simulink model "ABS_default"  (R2020b)
settings: Solver=VariableStepAuto  StartTime=0.0  StopTime=60.0  RelTol=1e-3
InitFcn:
  | T_B = 0.1;
  | J = 1.13;
  | g = 9.81;
  | road_coeff = [
  |                 1.2801 23.990 0.5200
  |                 0.8570 33.822 0.3470
  |                 1.1973 25.168 0.5373
  |                 0.4004 33.708 0.1204
  |                 0.1946 94.129 0.0646
  |                 0.0500 306.39 0.0010
  |               ];
  | load('ANFIS.mat','train_fis');
  | ce = road_coeff(sel,:);
values from neighbouring files (symbols this model uses):
  Kpid = actSelGen(i,:)    [ABS_ga.m]    (also in ABS_pso.m = Swarm.Particles(k).X)
undefined symbols (not defined in the file or in its folder): m, R, v_x
libraries: fuzblock x1, pid_lib x1
settings Model: Creator=hadlaczkyb  LastModifiedBy=hadlaczkyb
settings DataIOCC: ReturnWorkspaceOutputs=off
settings DebuggingCC: ArithmeticOperatorsInVariantConditions=warning
settings SFSimCC: SimUseLocalCustomCode=off  CustomCodeUndefinedFunction=UseInterfaceOnly
settings RTWCC: RTWUseLocalCustomCode=off

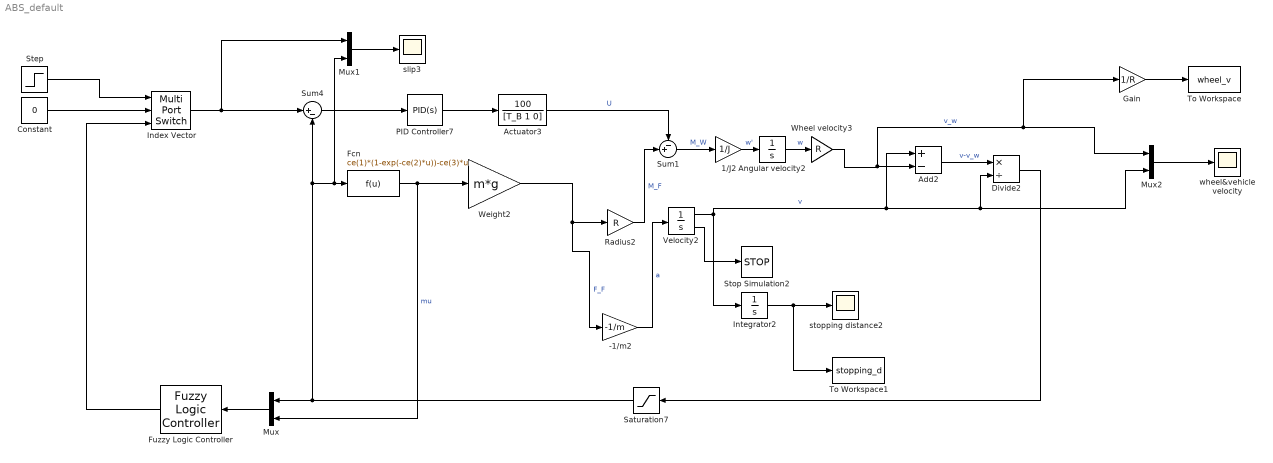
== system ABS_default ==
  -1/m2 : Gain  Gain=-1/m
  1/J2 : Gain  Gain=1/J
  Actuator3 : TransferFcn  Numerator=[0 0 100]  Denominator=[T_B 1 0]
  Add2 : Sum  Inputs=+-
  Angular velocity2 : Integrator  InitialCondition=v_x/R  LimitOutput=on  UpperSaturationLimit=1000  LowerSaturationLimit=0
  Constant : Constant  Value=0
  Divide2 : Product  Inputs=*/
  Fcn : Fcn  Expr=ce(1)*(1-exp(-ce(2)*u))-ce(3)*u
  Fuzzy Logic Controller : fuzblock/Fuzzy Logic  Controller  FIS=train_fis  OutputSampleNumber=101  DataType=double  FuzzifiedInputs=off  RuleFiringStrengths=off  RuleOutputs=off  AggregatedOutputs=off  SimulateUsing=Interpreted execution  OutOfRangeInputValueMessage=warning  NoRuleFiredMessage=warning  EmptyOutputFuzzySetMessage=warning
  Gain : Gain  Gain=1/R
  Index Vector : MultiPortSwitch  DataPortOrder=Zero-based contiguous  Inputs=2  zeroidx=on
  Integrator2 : Integrator
  Mux : Mux  Inputs=2
  Mux1 : Mux  Inputs=2
  Mux2 : Mux  Inputs=2
  PID Controller7 : pid_lib/PID Controller  Controller=PID  Form=Parallel  TimeDomain=Continuous-time  UseExternalTs=off  SampleTime=-1  IntegratorMethod=Forward Euler  FilterMethod=Forward Euler  ControllerParametersSource=internal  P=Kpid(1)  I=Kpid(2)  D=Kpid(3)  UseFilter=on  N=1000  TunerSelectOption=Transfer Function Based (PID Tuner App)  InitialConditionSource=internal  InitialConditionForIntegrator=0  InitialConditionForFilter=0  DifferentiatorICPrevScaledInput=0  ExternalReset=none  TrackingMode=off  Kt=1  LimitOutput=off  SatLimitsSource=internal  UpperSaturationLimit=inf  LowerSaturationLimit=-inf  LinearizeAsGain=on  AntiWindupMode=none  Kb=1  POutMin=[]  POutMax=[]  IOutMin=[]  IOutMax=[]  DOutMin=[]  DOutMax=[]  NOutMin=[]  NOutMax=[]  SumOutMin=[]  SumOutMax=[]  SaturationOutMin=[]  SaturationOutMax=[]  PParamMin=[]  PParamMax=[]  IParamMin=[]  IParamMax=[]  DParamMin=[]  DParamMax=[]  NParamMin=[]  NParamMax=[]  KbParamMin=[]  KbParamMax=[]  KtParamMin=[]  KtParamMax=[]  KbOutMin=[]  KbOutMax=[]  KtOutMin=[]  KtOutMax=[]  IntegratorOutMin=[]  IntegratorOutMax=[]  FilterOutMin=[]  FilterOutMax=[]  SumI1OutMin=[]  SumI1OutMax=[]  SumI2OutMin=[]  SumI2OutMax=[]  SumI3OutMin=[]  SumI3OutMax=[]  SumI4OutMin=[]  SumI4OutMax=[]  SumDOutMin=[]  SumDOutMax=[]  DifferentiatorOutMin=[]  DifferentiatorOutMax=[]  FilterDiffOutCoefMin=[]  FilterDiffOutCoefMax=[]  ReciprocalOutMin=[]  ReciprocalOutMax=[]  SumDenOutMin=[]  SumDenOutMax=[]  SumNumOutMin=[]  SumNumOutMax=[]  DivideOutMin=[]  DivideOutMax=[]  UdiffTsProdOutMin=[]  UdiffTsProdOutMax=[]  NTsProdOutMin=[]  NTsProdOutMax=[]  UintegralTsProdOutMin=[]  UintegralTsProdOutMax=[]  UngainTsProdOutMin=[]  UngainTsProdOutMax=[]  IntegratorContinuousStateAttributes=''  IntegratorStateMustResolveToSignalObject=off  IntegratorRTWStateStorageClass=Auto  FilterContinuousStateAttributes=''  FilterStateMustResolveToSignalObject=off  FilterRTWStateStorageClass=Auto  ParallelPVariant=InternalParameters  IdealPVariant=Disabled  IVariant=InternalParameters  DVariant=InternalParameters  IntegratorVariant=Continuous  SatVariant=Disabled  AWVariant=Passthrough  PCopyVariant=Disabled  TRVariant=Disabled  FdbkBlocksVariant=Forward  IdealPFdbkVariant=Disabled  SatFdbkVariant=Disabled  DerivativeFilterVariant=ContFilter  NVariant=InternalParameters  NCopyVariant=Disabled  FilterICVariant=InternalICsFilter  IntegratorICVariant=InternalICs  ExternalResetVariant=Disabled  TRSumVariant=Passthrough  SumFdbkVariant=Disabled  SumVariant=Sum_PID  TsampFilterVariant=InternalTs  TsampNgainVariant=Passthrough  TsampIntegralVariant=Passthrough  ExternalSaturationOutDataTypeStr=Inherit: Same as second input
  Radius2 : Gain  Gain=R
  Saturation7 : Saturate  UpperLimit=1  LowerLimit=0
  Step : Step  Time=5  SampleTime=0
  Stop Simulation2 : Stop
  Sum1 : Sum  Inputs=-+|
  Sum4 : Sum  Inputs=|+-
  To Workspace : ToWorkspace  VariableName=wheel_v  SaveFormat=Timeseries  SampleTime=-1
  To Workspace1 : ToWorkspace  VariableName=stopping_d  SaveFormat=Timeseries  SampleTime=-1
  Velocity2 : Integrator  InitialCondition=v_x  LimitOutput=on  UpperSaturationLimit=1000  LowerSaturationLimit=1  ShowSaturationPort=on
  Weight2 : Gain  Gain=m*g
  Wheel velocity3 : Gain  Gain=R
  slip3 : Scope
  stopping distance2 : Scope
  wheel&vehicle velocity : Scope
  wires:
  Mux2/1 -> wheel&vehicle velocity/1
  Constant/1 -> Index Vector/2
  Step/1 -> Index Vector/1
  Fcn/1 -> Weight2/1, Mux/2  "mu"
  Velocity2/2 -> Stop Simulation2/1
  Weight2/1 -> -1/m2/1, Radius2/1  "F_F"
  1/J2/1 -> Angular velocity2/1  "w'"
  Sum4/1 -> PID Controller7/1
  Add2/1 -> Divide2/1  "v-v_w"
  Sum1/1 -> 1/J2/1  "M_W"
  Angular velocity2/1 -> Wheel velocity3/1  "w"
  Velocity2/1 -> Integrator2/1, Divide2/2, Mux2/2, Add2/1  "v"
  Radius2/1 -> Sum1/2  "M_F"
  Integrator2/1 -> To Workspace1/1, stopping distance2/1
  Mux/1 -> Fuzzy Logic Controller/1
  PID Controller7/1 -> Actuator3/1
  Fuzzy Logic Controller/1 -> Index Vector/3
  Mux1/1 -> slip3/1
  Actuator3/1 -> Sum1/1  "U"
  Saturation7/1 -> Mux1/2, Fcn/1, Sum4/2, Mux/1
  Divide2/1 -> Saturation7/1
  -1/m2/1 -> Velocity2/1  "a"
  Index Vector/1 -> Sum4/1, Mux1/1
  Wheel velocity3/1 -> Add2/2, Gain/1, Mux2/1  "v_w"
  Gain/1 -> To Workspace/1
